simulink library "ForcesAndMoments_Lib"  (R2016b)
settings: Solver=VariableStepAuto  StartTime=0.0  StopTime=10.0  RelTol=1e-3
values from neighbouring files (symbols this model uses):
  AC =     [UAV_modelconfig.mat]
undefined symbols (not defined in the file or in its folder): TrimCondition
libraries: OpenFlightUtilLib x3
settings Model: Creator=UAVLAB  LastModifiedBy=UAVLAB

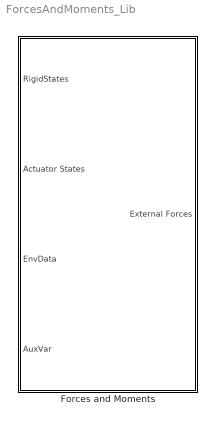
== system ForcesAndMoments_Lib ==
  Forces and Moments : Subsystem

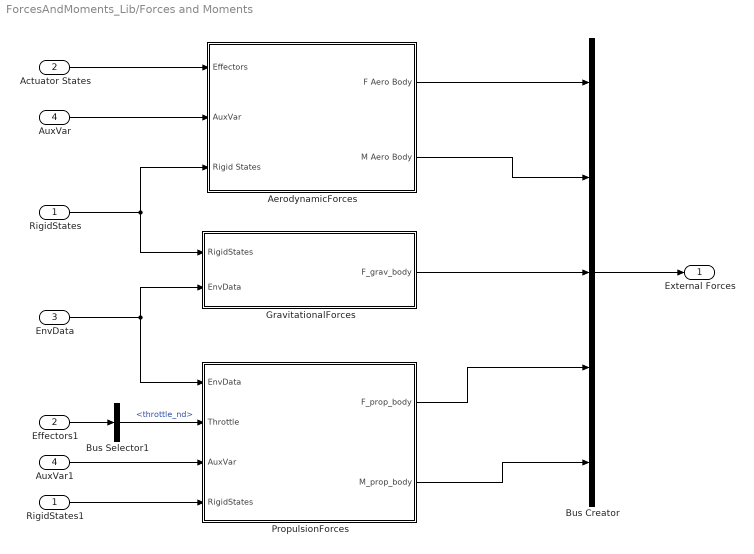
== system ForcesAndMoments_Lib/Forces and Moments ==
  RigidStates : Inport  OutDataTypeStr=Bus: RigidStates
  Actuator States : Inport  Port=2  OutDataTypeStr=Bus: Effectors
  EnvData : Inport  Port=3  OutDataTypeStr=Bus: EnvData
  AuxVar : Inport  Port=4  OutDataTypeStr=Bus: AuxVar
  AerodynamicForces : Subsystem
  AuxVar1 : InportShadow  Port=4  OutDataTypeStr=Bus: AuxVar
  Bus Selector1 : BusSelector  OutputSignals=Motor.throttle_nd
  Bus Creator : BusCreator  Inputs=5
  Effectors1 : InportShadow  Port=2  OutDataTypeStr=Bus: Effectors
  "GravitationalForces " : Subsystem
  PropulsionForces : Subsystem
  RigidStates1 : InportShadow  OutDataTypeStr=Bus: RigidStates
  External Forces : Outport
  wires:
  PropulsionForces/2(M_prop_body) -> Bus Creator/5
  PropulsionForces/1(F_prop_body) -> Bus Creator/4
  AerodynamicForces/1(F Aero Body) -> Bus Creator/1
  AerodynamicForces/2(M Aero Body) -> Bus Creator/2
  AuxVar1/1 -> PropulsionForces/3(AuxVar)
  RigidStates/1 -> AerodynamicForces/3(Rigid States), "GravitationalForces "/1(RigidStates)
  AuxVar/1 -> AerodynamicForces/2(AuxVar)
  Bus Creator/1 -> External Forces/1
  "GravitationalForces "/1(F_grav_body) -> Bus Creator/3
  RigidStates1/1 -> PropulsionForces/4(RigidStates)
  Bus Selector1/1 -> PropulsionForces/2(Throttle)  "<throttle_nd>"
  EnvData/1 -> "GravitationalForces "/2(EnvData), PropulsionForces/1(EnvData)
  Effectors1/1 -> Bus Selector1/1
  Actuator States/1 -> AerodynamicForces/1(Effectors)

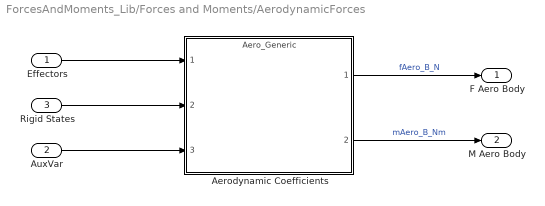
== system ForcesAndMoments_Lib/Forces and Moments/AerodynamicForces ==
  Effectors : Inport  OutDataTypeStr=Bus: Effectors
  AuxVar : Inport  Port=2
  Rigid States : Inport  Port=3  OutDataTypeStr=Bus: RigidStates
  Aerodynamic Coefficients : ModelReference  ModelNameDialog=Aero_Generic  SimulationMode=Normal  Variant=on  ModelReferenceVersion=1.53
  F Aero Body : Outport
  M Aero Body : Outport  Port=2
  wires:
  Aerodynamic Coefficients/1 -> F Aero Body/1  "fAero_B_N"
  Aerodynamic Coefficients/2 -> M Aero Body/1  "mAero_B_Nm"
  Effectors/1 -> Aerodynamic Coefficients/1
  AuxVar/1 -> Aerodynamic Coefficients/3
  Rigid States/1 -> Aerodynamic Coefficients/2

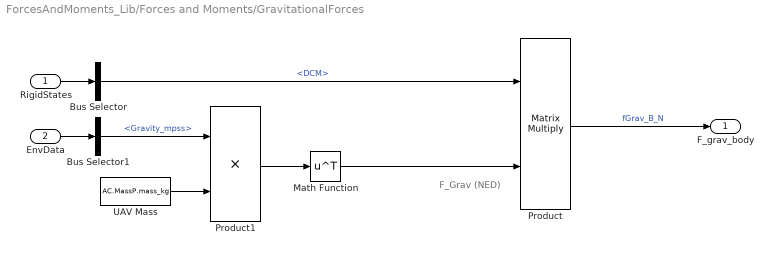
== system ForcesAndMoments_Lib/Forces and Moments/GravitationalForces  ==
  note: F_Grav (NED)
  RigidStates : Inport  OutDataTypeStr=Bus: RigidStates
  EnvData : Inport  Port=2  OutDataTypeStr=Bus: EnvData
  Bus Selector : BusSelector  OutputSignals=DCM
  Bus Selector1 : BusSelector  OutputSignals=Gravity_mpss
  Math Function : Math  Operator=transpose  SaturateOnIntegerOverflow=on
  Product : Product  Multiplication=Matrix(*)  SaturateOnIntegerOverflow=on  RndMeth=Zero  InputSameDT=on  OutDataTypeStr=Inherit: Same as first input
  Product1 : Product  SaturateOnIntegerOverflow=on  RndMeth=Zero  InputSameDT=on  OutDataTypeStr=Inherit: Same as first input
  UAV Mass : Constant  Value=AC.MassP.mass_kg
  F_grav_body : Outport
  wires:
  Product/1 -> F_grav_body/1  "fGrav_B_N"
  Bus Selector/1 -> Product/1  "<DCM>"
  RigidStates/1 -> Bus Selector/1
  EnvData/1 -> Bus Selector1/1
  Bus Selector1/1 -> Product1/1  "<Gravity_mpss>"
  UAV Mass/1 -> Product1/2
  Product1/1 -> Math Function/1
  Math Function/1 -> Product/2

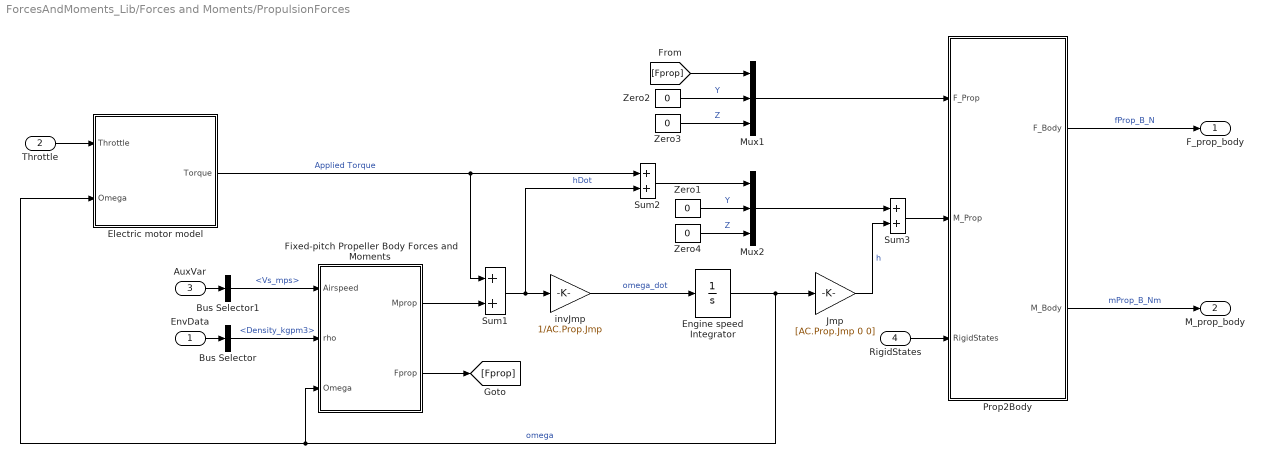
== system ForcesAndMoments_Lib/Forces and Moments/PropulsionForces ==
  EnvData : Inport  OutDataTypeStr=Bus: EnvData
  Throttle : Inport  Port=2  OutDataTypeStr=double
  AuxVar : Inport  Port=3  OutDataTypeStr=Bus: AuxVar
  RigidStates : Inport  Port=4  OutDataTypeStr=Bus: RigidStates
  Bus Selector : BusSelector  OutputSignals=Density_kgpm3
  Bus Selector1 : BusSelector  OutputSignals=WindAxesParams.Vs_mps
  Electric motor model : Subsystem
  Engine speed Integrator : Integrator  InitialCondition=TrimCondition.EngineSpeedIni  LimitOutput=on  UpperSaturationLimit=AC.Prop.OmegaSaturation.Upper  LowerSaturationLimit=AC.Prop.OmegaSaturation.Lower
  Fixed-pitch Propeller Body Forces and Moments : Subsystem
  Jmp : Gain  Gain=[AC.Prop.Jmp 0 0]  SaturateOnIntegerOverflow=on  OutDataTypeStr=Inherit: Same as input  ParamDataTypeStr=Inherit: Same as input
  Mux1 : Mux  Inputs=3
  Mux2 : Mux  Inputs=3
  Prop2Body : Subsystem
  Sum1 : Sum  SaturateOnIntegerOverflow=on  InputSameDT=on  OutDataTypeStr=Inherit: Same as first input
  Sum2 : Sum
  Sum3 : Sum
  Zero{1..4} (4 alike) : Constant  Value=0
  invJmp : Gain  Gain=1/AC.Prop.Jmp
  F_prop_body : Outport
  M_prop_body : Outport  Port=2
  wires:
  RigidStates/1 -> Prop2Body/3(RigidStates)
  Prop2Body/1(F_Body) -> F_prop_body/1  "fProp_B_N"
  Sum3/1 -> Prop2Body/2(M_Prop)
  Mux2/1 -> Sum3/1
  Sum2/1 -> Mux2/1
  Zero1/1 -> Mux2/2  "Y"
  Zero4/1 -> Mux2/3  "Z"
  Mux1/1 -> Prop2Body/1(F_Prop)
  Jmp/1 -> Sum3/2  "h"
  Fixed-pitch Propeller Body Forces and Moments/2(Fprop) -> [Fprop]
  Fixed-pitch Propeller Body Forces and Moments/1(Mprop) -> Sum1/2
  Bus Selector/1 -> Fixed-pitch Propeller Body Forces and Moments/2(rho)  "<Density_kgpm3>"
  Bus Selector1/1 -> Fixed-pitch Propeller Body Forces and Moments/1(Airspeed)  "<Vs_mps>"
  [Fprop] -> Mux1/1
  Prop2Body/2(M_Body) -> M_prop_body/1  "mProp_B_Nm"
  AuxVar/1 -> Bus Selector1/1
  EnvData/1 -> Bus Selector/1
  Zero2/1 -> Mux1/2  "Y"
  Zero3/1 -> Mux1/3  "Z"
  Engine speed Integrator/1 -> Jmp/1, Fixed-pitch Propeller Body Forces and Moments/3(Omega), Electric motor model/2(Omega)  "omega"
  Electric motor model/1(Torque) -> Sum2/1, Sum1/1  "Applied Torque"
  Throttle/1 -> Electric motor model/1(Throttle)
  Sum1/1 -> Sum2/2, invJmp/1  "hDot"
  invJmp/1 -> Engine speed Integrator/1  "omega_dot"

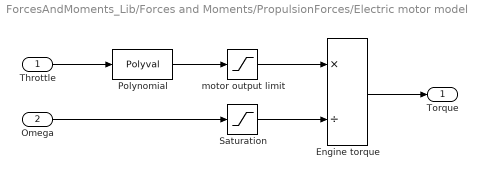
== system ForcesAndMoments_Lib/Forces and Moments/PropulsionForces/Electric motor model ==
  Throttle : Inport  OutDataTypeStr=double
  Omega : Inport  Port=2  OutDataTypeStr=double
  Engine torque : Product  Inputs=*/  SaturateOnIntegerOverflow=on  InputSameDT=on  OutDataTypeStr=Inherit: Same as first input
  Polynomial : Polyval  Coefs=AC.Prop.Power
  Saturation : Saturate  UpperLimit=AC.Prop.OmegaSaturation.Upper  LowerLimit=AC.Prop.OmegaSaturation.Lower
  motor output limit : Saturate  UpperLimit=AC.Prop.ThrottleOutputLimit.Upper  LowerLimit=AC.Prop.ThrottleOutputLimit.Lower
  Torque : Outport
  wires:
  motor output limit/1 -> Engine torque/1
  Throttle/1 -> Polynomial/1
  Polynomial/1 -> motor output limit/1
  Omega/1 -> Saturation/1
  Engine torque/1 -> Torque/1
  Saturation/1 -> Engine torque/2

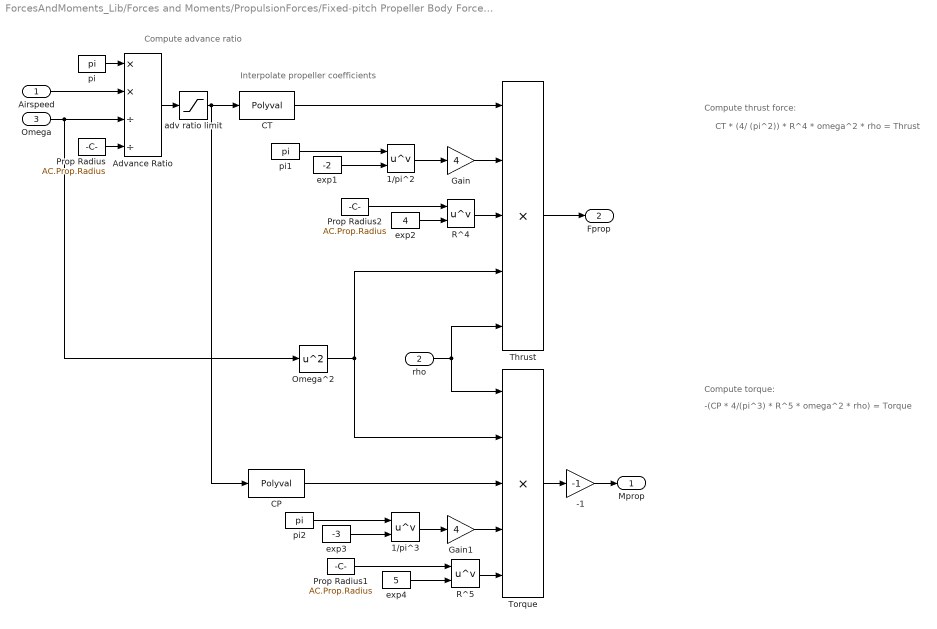
== system ForcesAndMoments_Lib/Forces and Moments/PropulsionForces/Fixed-pitch Propeller Body Forces and Moments ==
  note: -(CP * 4/(pi^3) * R^5 * omega^2 * rho) = Torque
  note: CT * (4/ (pi^2)) * R^4 * omega^2 * rho = Thrust
  note: Compute advance ratio
  note: Compute thrust force:
  note: Interpolate propeller coefficients
  note: Compute torque:
  Airspeed : Inport  OutDataTypeStr=double
  rho : Inport  Port=2  OutDataTypeStr=double
  Omega : Inport  Port=3  OutDataTypeStr=double
  -1 : Gain  Gain=-1  SaturateOnIntegerOverflow=on  OutDataTypeStr=Inherit: Same as input  ParamDataTypeStr=Inherit: Same as input
  1/pi^2 : Math  Operator=pow  SaturateOnIntegerOverflow=on
  1/pi^3 : Math  Operator=pow  SaturateOnIntegerOverflow=on
  Advance Ratio : Product  Inputs=**//  SaturateOnIntegerOverflow=on  InputSameDT=on  OutDataTypeStr=Inherit: Same as first input
  CP : Polyval  Coefs=AC.Prop.CP
  CT : Polyval  Coefs=AC.Prop.CT
  Gain : Gain  Gain=4  SaturateOnIntegerOverflow=on  OutDataTypeStr=Inherit: Same as input  ParamDataTypeStr=Inherit: Same as input
  Gain1 : Gain  Gain=4  SaturateOnIntegerOverflow=on  OutDataTypeStr=Inherit: Same as input  ParamDataTypeStr=Inherit: Same as input
  Omega^2 : Math  Operator=square  SaturateOnIntegerOverflow=on
  Prop Radius : Constant  Value=AC.Prop.Radius
  Prop Radius1 : Constant  Value=AC.Prop.Radius
  Prop Radius2 : Constant  Value=AC.Prop.Radius
  R^4 : Math  Operator=pow  SaturateOnIntegerOverflow=on
  R^5 : Math  Operator=pow  SaturateOnIntegerOverflow=on
  Thrust : Product  Inputs=5  SaturateOnIntegerOverflow=on  InputSameDT=on  OutDataTypeStr=Inherit: Same as first input
  Torque : Product  Inputs=5  SaturateOnIntegerOverflow=on  InputSameDT=on  OutDataTypeStr=Inherit: Same as first input
  adv ratio limit : Saturate  UpperLimit=0.7  LowerLimit=0
  exp1 : Constant  Value=-2
  exp2 : Constant  Value=4
  exp3 : Constant  Value=-3
  exp4 : Constant  Value=5
  pi : Constant  Value=pi
  pi1 : Constant  Value=pi
  pi2 : Constant  Value=pi
  Mprop : Outport
  Fprop : Outport  Port=2
  wires:
  adv ratio limit/1 -> CP/1, CT/1
  -1/1 -> Mprop/1
  pi/1 -> Advance Ratio/1
  pi2/1 -> 1/pi^3/1
  Prop Radius2/1 -> R^4/1
  Prop Radius1/1 -> R^5/1
  exp1/1 -> 1/pi^2/2
  Airspeed/1 -> Advance Ratio/2
  rho/1 -> Torque/1, Thrust/5
  Omega/1 -> Advance Ratio/3, Omega^2/1
  pi1/1 -> 1/pi^2/1
  Prop Radius/1 -> Advance Ratio/4
  Advance Ratio/1 -> adv ratio limit/1
  Omega^2/1 -> Torque/2, Thrust/4
  exp3/1 -> 1/pi^3/2
  1/pi^2/1 -> Gain/1
  1/pi^3/1 -> Gain1/1
  exp2/1 -> R^4/2
  R^4/1 -> Thrust/3
  exp4/1 -> R^5/2
  R^5/1 -> Torque/5
  Gain/1 -> Thrust/2
  Gain1/1 -> Torque/4
  Thrust/1 -> Fprop/1
  Torque/1 -> -1/1
  CT/1 -> Thrust/1
  CP/1 -> Torque/3

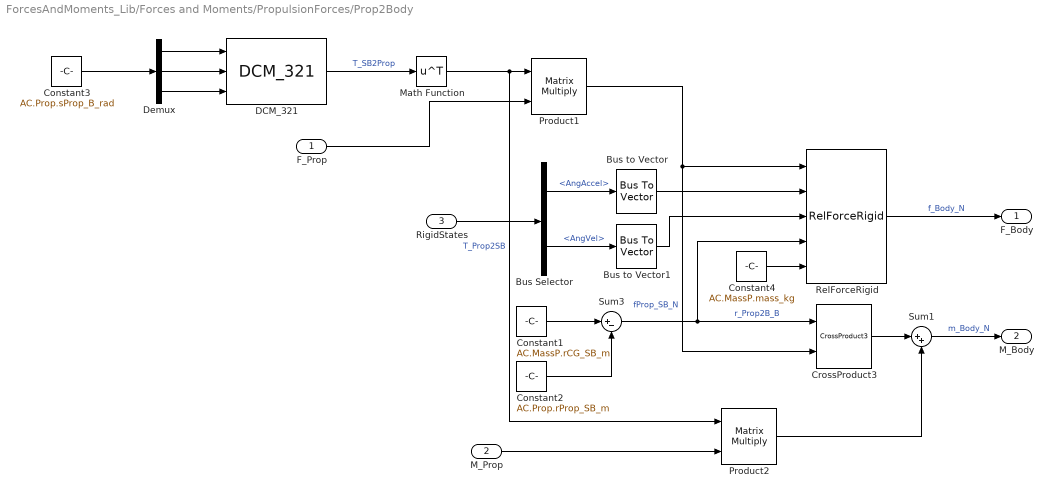
== system ForcesAndMoments_Lib/Forces and Moments/PropulsionForces/Prop2Body ==
  F_Prop : Inport
  M_Prop : Inport  Port=2
  RigidStates : Inport  Port=3
  Bus Selector : BusSelector  OutputSignals=AngAccel,AngVel
  Bus to Vector : BusToVector
  Bus to Vector1 : BusToVector
  Constant1 : Constant  Value=AC.MassP.rCG_SB_m
      settings: AttributesFormatString=%<Value>
  Constant2 : Constant  Value=AC.Prop.rProp_SB_m
      settings: AttributesFormatString=%<Value>
  Constant3 : Constant  Value=AC.Prop.sProp_B_rad
      settings: AttributesFormatString=%<Value>
  Constant4 : Constant  Value=AC.MassP.mass_kg
      settings: AttributesFormatString=%<Value>
  CrossProduct3 : OpenFlightUtilLib/Math/CrossProduct3
  DCM_321 : OpenFlightUtilLib/Transformations/DCM_321
  Demux : Demux  Outputs=3
  Math Function : Math  Operator=transpose  SaturateOnIntegerOverflow=on
  Product1 : Product  Multiplication=Matrix(*)  RndMeth=Zero
  Product2 : Product  Multiplication=Matrix(*)  RndMeth=Zero
  RelForceRigid : OpenFlightUtilLib/Kinematics and Dynamics/RelForceRigid
  Sum1 : Sum  Inputs=|++  SaturateOnIntegerOverflow=on
  Sum3 : Sum  Inputs=|+-  SaturateOnIntegerOverflow=on
  F_Body : Outport
  M_Body : Outport  Port=2
  wires:
  Constant4/1 -> RelForceRigid/5
  Product2/1 -> Sum1/2
  DCM_321/1 -> Math Function/1  "T_SB2Prop"
  Demux/2 -> DCM_321/2
  Demux/1 -> DCM_321/1
  Demux/3 -> DCM_321/3
  Constant3/1 -> Demux/1
  Sum1/1 -> M_Body/1  "m_Body_N"
  CrossProduct3/1 -> Sum1/1
  M_Prop/1 -> Product2/2
  RelForceRigid/1 -> F_Body/1  "f_Body_N"
  RigidStates/1 -> Bus Selector/1
  Sum3/1 -> RelForceRigid/4, CrossProduct3/1  "r_Prop2B_B"
  Product1/1 -> CrossProduct3/2, RelForceRigid/1  "fProp_SB_N"
  Math Function/1 -> Product1/1, Product2/1  "T_Prop2SB"
  F_Prop/1 -> Product1/2
  Bus Selector/2 -> Bus to Vector1/1  "<AngVel>"
  Bus to Vector1/1 -> RelForceRigid/3
  Bus to Vector/1 -> RelForceRigid/2
  Bus Selector/1 -> Bus to Vector/1  "<AngAccel>"
  Constant2/1 -> Sum3/2
  Constant1/1 -> Sum3/1
